simulink model "filtro_kalman"  (R2012b)
settings: Solver=ode3  StartTime=0.0  StopTime=10  FixedStep=1e-4  RelTol=1e-3
undefined symbols (not defined in the file): A, B, C
libraries: simulink x2, Encoder x1
settings Model: Creator=h3now  LastModifiedBy=h3now

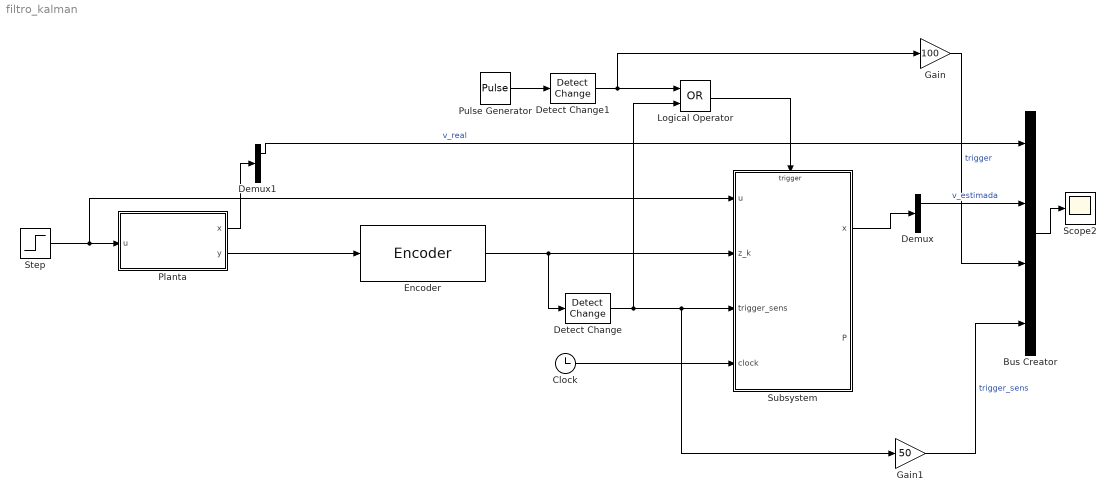
== system filtro_kalman ==
  Bus Creator : BusCreator
  Clock : Clock
  Demux : Demux  Outputs=2
  Demux1 : Demux  Outputs=2
  Detect Change : simulink/Logic and Bit Operations/Detect Change  vinit=0  InputProcessing=Inherited  OutDataTypeStr=boolean
  Detect Change1 : simulink/Logic and Bit Operations/Detect Change  vinit=0  InputProcessing=Inherited  OutDataTypeStr=boolean
  Encoder : Encoder/Encoder  Nr=3
  Gain : Gain  Gain=100  OutDataTypeStr=double
  Gain1 : Gain  Gain=50  OutDataTypeStr=double
  Logical Operator : Logic  Operator=OR  AllPortsSameDT=off  OutDataTypeStr=boolean
  Planta : Subsystem
  Pulse Generator : DiscretePulseGenerator  PulseType=Time based  Period=0.3  PulseWidth=50
  Scope2 : Scope
      settings: ShowLegends=on  YMin=-250  YMax=100
  Step : Step  Time=5  Before=5  After=-5  SampleTime=0
  Subsystem : Subsystem
  wires:
  Planta/2(y) -> Encoder/1
  Encoder/1 -> Detect Change/1, Subsystem/2("z_k ")
  Step/1 -> Subsystem/1(u), Planta/1(u)
  Demux/1 -> Bus Creator/2  "v_estimada"
  Planta/1(x) -> Demux1/1
  Demux1/1 -> Bus Creator/1  "v_real"
  Bus Creator/1 -> Scope2/1
  Detect Change/1 -> Logical Operator/2, Gain1/1, Subsystem/3(trigger_sens)
  Clock/1 -> Subsystem/4(clock)
  Subsystem/1(x) -> Demux/1
  Pulse Generator/1 -> Detect Change1/1
  Detect Change1/1 -> Gain/1, Logical Operator/1
  Logical Operator/1 -> Subsystem/Trigger
  Gain/1 -> Bus Creator/3  "trigger"
  Gain1/1 -> Bus Creator/4  "trigger_sens"

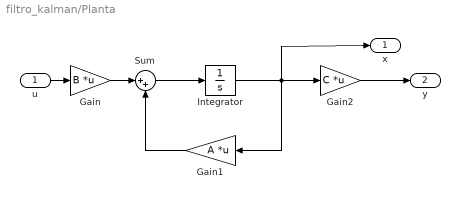
== system filtro_kalman/Planta ==
  u : Inport
  Gain : Gain  Gain=B  Multiplication=Matrix(K*u)
  Gain1 : Gain  Gain=A  Multiplication=Matrix(K*u)
  Gain2 : Gain  Gain=C  Multiplication=Matrix(K*u)
  Integrator : Integrator
  Sum : Sum  Inputs=|++
  x : Outport
  y : Outport  Port=2
  wires:
  u/1 -> Gain/1
  Integrator/1 -> x/1, Gain2/1, Gain1/1
  Gain2/1 -> y/1
  Sum/1 -> Integrator/1
  Gain1/1 -> Sum/2
  Gain/1 -> Sum/1

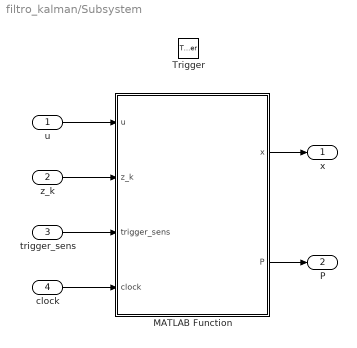
== system filtro_kalman/Subsystem ==
  u : Inport
  "z_k " : Inport  Port=2
  trigger_sens : Inport  Port=3
  clock : Inport  Port=4
  Trigger : TriggerPort  PortDimensions=1
  MATLAB Function : MATLAB Function  TreatAsAtomicUnit=on
  x : Outport
  P : Outport  Port=2
  wires:
  MATLAB Function/1(x) -> x/1
  MATLAB Function/2(P) -> P/1
  trigger_sens/1 -> MATLAB Function/3(trigger_sens)
  u/1 -> MATLAB Function/1(u)
  clock/1 -> MATLAB Function/4(clock)
  "z_k "/1 -> MATLAB Function/2(z_k)

== matlab function filtro_kalman/Subsystem/MATLAB Function ==
  data: u input; z_k input; x output; trigger_sens input; P output; clock input
function [x,P] = fcn(u, z_k, trigger_sens, clock)
%#codegen

persistent t_old;
persistent x_posteriori_old;
persistent P_posteriori_old;

if( isempty(t_old) || isempty(x_posteriori_old) || isempty(P_posteriori_old) )
    t_old = 0;
    x_posteriori_old = [0 0]';
    P_posteriori_old = [10 0; 0 10];
end


deltaT = clock - t_old;
F = [1-0.2*deltaT 0 ; deltaT 1];
B = [10*deltaT ; 0];
H = [0 1];
Q = eye(2)*0.6;
R = eye(1)*0.2;

% Previsão
x_priori = F * x_posteriori_old + B*u;
P_priori = F * P_posteriori_old * F' + Q;

% Atualização
if(trigger_sens == 1)
    y_tilde = z_k - H * x_priori;
    S = H * P_priori * H' + R;
    K = P_priori * H' / S;
    x_posteriori = x_priori + K * y_tilde;
    P_posteriori = (eye(size(K*H)) * K * H) * P_priori;
else
    x_posteriori = x_priori;
    P_posteriori = P_priori;
end

x = x_posteriori;
P = P_posteriori;

x_posteriori_old = x_posteriori;
P_posteriori_old = P_posteriori;
t_old = clock;
